simulink model "generic_20231123_1032"  (R2022b)
settings: Solver=ode45  StartTime=0.0  StopTime=50  RelTol=1e-3  EnableMultiTasking=on
model workspace (MAT data in the model file):
  A = 1
  B = 1.19071237887
  kd = -9.99955278144
  ki = 0.00519416981022
  kp = 9.99999979837
undefined symbols (not defined in the file): brake_select, curvature, DiscIntNeverNeededParam, speed
libraries: CarMaker4SL x88, simulink x1, mpcadaslib x1
(part 1 of 4)
settings Model: Creator=fh  LastModifiedBy=Admin
settings SolverCC: AlgebraicLoopSolver=TrustRegion
settings DataIOCC: LimitDataPoints=on  SaveFormat=Array  SignalLoggingSaveFormat=ModelDataLogs  ReturnWorkspaceOutputs=off  SignalLoggingName=sigsOut
settings OptimizationCC: BooleanDataType=off  ExpressionDepthLimit=2147483647  InitFltsAndDblsToZero=on  LifeSpan=inf
settings DebuggingCC: SaveWithParameterizedLinksMsg=none  UnderspecifiedInitializationDetection=Classic  MergeDetectMultiDrivingBlocksExec=none  SignalResolutionControl=TryResolveAllWithWarning  MultiTaskDSMMsg=warning  MultiTaskCondExecSysMsg=none  FcnCallInpInsideContextMsg=warning  UnconnectedInputMsg=warning  UnconnectedOutputMsg=warning  UnconnectedLineMsg=warning  StateNameClashWarn=warning  SFUnexpectedBacktrackingDiag=warning  SFNoUnconditionalDefaultTransitionDiag=warning  SFMachineParentedDataDiag=warning  ArithmeticOperatorsInVariantConditions=warning
settings HardwareCC: ProdBitPerPointer=32  ProdBitPerSizeT=32  ProdBitPerPtrDiffT=32  ProdLargestAtomicFloat=None  ProdIntDivRoundTo=Undefined  ProdEndianess=Unspecified  ProdWordSize=32  ProdHWDeviceType=32-bit Generic  TargetUnknown=on
settings ModelReferenceCC: EnableRefExpFcnMdlSchedulingChecks=on  PropagateSignalLabelsOutOfModel=off
settings SFSimCC: SimUseLocalCustomCode=off  CustomCodeUndefinedFunction=UseInterfaceOnly
settings RTWCC: RTWUseLocalCustomCode=off
settings CodeAppCC: MaxIdLength=63  StateflowObjectComments=on
settings GRTTargetCC: TargetFcnLib=ansi_tfl_tmw.mat  TargetLangStandard=C89/C90 (ANSI)  CombineOutputUpdateFcns=off  GRTInterface=on
settings ConfigComp: CovMetricSettings=dw  CovSaveCumulativeToWorkspaceVar=on  CovSaveSingleToWorkspaceVar=on  CovExternalEMLEnable=off

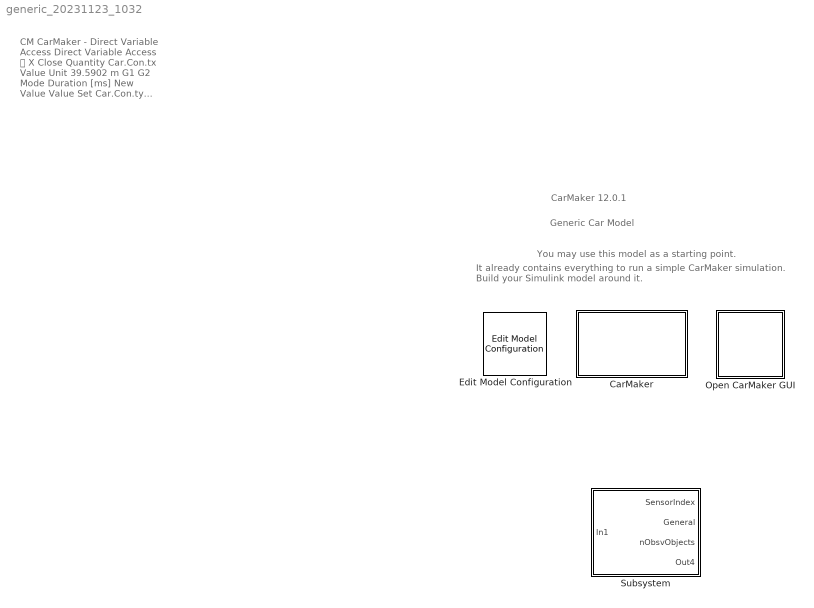
== system generic_20231123_1032 ==
  note: CM CarMaker - Direct Variable Access
      | Direct Variable Access
      | ப
      | X
      | Close
      | Quantity
      | Car.Con.tx
      | Value Unit 39.5902 m
      | G1 G2 Mode Duration [ms] New Value
      | Value
      | Set
      | Car.Con.ty
      | 503.638 m
      | Value
      | Set
      | Car.Con.tz
      | 12.6573 m
      | Value
      | Set
      | Car Road Path.DevAng
      | -0.0358446 rad
      | Value
      | Set
      | Car.Road.tx
      | 40.1728 m
      | Value
      | Set
      | Car Road.Path.DevDist
      | -0.152703 m
      | Ε
      | Value
      | Set
      | AccelCtrl.ACC.DesiredSpd
      | 31.2619 m/s
      | Value
      | Set
      | Sensor.Road.VehSensor_0.Path.tx
      | Sensor.Road.VehSensor_0.Path.ty
      | 0 m
      | Value
      | Set
      | 0 m
      | Value
      | Set
      | Sensor.Road.VehSensor_0.Path.tz
      | 0 m
      | Value
      | Set
      | Set Group 1
      | Set Group 2
      | Release all
  note: Generic Car Model
  note: You may use this model as a starting point.
  note: It already contains everything to run a simple CarMaker simulation.
      | Build your Simulink model around it.
  note: CarMaker 12.0.1
  CarMaker : Subsystem  TreatAsAtomicUnit=on
      mask Display: image(imread('CarMakerSys.png'));
  Edit Model Configuration : CarMaker4SL/Edit Model Configuration  SFunctionModules=''
  Open CarMaker GUI : Subsystem  LoadFcn=if ~length(which('cmself')), cmenv; end
      settings: OpenFcn=cmblockmagic('gui_fix_display'); CM_Simulink
      mask Display: image(imread('CarMakerGUI.png'));
  Subsystem : Subsystem

== system generic_20231123_1032/CarMaker ==
  CM_FIRST : Subsystem
  CM_LAST : Subsystem
  DrivMan : Subsystem
  Ground : Ground
  IPG Vehicle : Subsystem
  Terminator : Terminator
  VehicleControl : Subsystem
  wires:
  DrivMan/2(DrivMan.Out) -> VehicleControl/2(DrivMan.In)
  DrivMan/1(Sync_Out) -> VehicleControl/1(Sync_In)
  CM_FIRST/2(Env.Misc) -> DrivMan/2(Env.Misc)
  CM_FIRST/1(Sync_Out) -> DrivMan/1(Sync_In)
  CM_LAST/1(Sync_Out) -> Terminator/1
  Ground/1 -> CM_FIRST/1(Sync_In)
  IPG Vehicle/1(Sync_Out) -> CM_LAST/1(Sync_In)
  VehicleControl/1(Sync_Out) -> IPG Vehicle/1(Sync_In)
  VehicleControl/3(VhclCtrl.Steering) -> IPG Vehicle/3(VhclCtrl.Steering)
  VehicleControl/4(Vhcl.Wheel.In) -> IPG Vehicle/4(Vhcl.Wheel.In)
  VehicleControl/5(Vhcl.Misc) -> IPG Vehicle/5(Vhcl.Misc)
  VehicleControl/6(VhclCtrl.Brake) -> IPG Vehicle/6(VhclCtrl.Brake)
  VehicleControl/7(VhclCtrl.PT) -> IPG Vehicle/7(VhclCtrl.PT)
  VehicleControl/2(Vhcl.Model.Source) -> IPG Vehicle/2(Vhcl.Model.Source)

== system generic_20231123_1032/Open CarMaker GUI ==
  S-Function : S-Function  FunctionName=cm_gui  SFunctionDeploymentMode=off  EnableBusSupport=off

== system generic_20231123_1032/Subsystem ==
  In1 : Inport
  ADASRP Receive : CarMaker4SL/ADASRP Receive  Commented=on  xstime=Continuous
      settings: SourceProductName=CarMaker4SL
  Bus Selector : BusSelector  Commented=on  OutputSignals=ObjID,Type,DrvOn,LengthRear,LengthFront,Width,tPathOff,InDrvDir,nObjF,nObjR
  Bus Selector1 : BusSelector  Commented=on  OutputSignals=DistToLeftBorder,DistToRightBorder
  Constant : Constant  Commented=on  Value=0
  Constant1 : Constant  Commented=on  Value=0
  Object Sensor : CarMaker4SL/Sensors/Object Sensor  Commented=on  xname=0  xstime=Inherited
      settings: SourceProductName=CarMaker4SL
  Radar Sensor : CarMaker4SL/Sensors/Radar Sensor  Commented=on  xname=0  xstime=Continuous
      settings: SourceProductName=CarMaker4SL
  Scope : Scope  Commented=on  NumInputPorts=2
  Scope1 : Scope  Commented=on
  Scope2 : Scope  Commented=on  NumInputPorts=10
  SensorIndex : Outport
  General : Outport  Port=2
  nObsvObjects : Outport  Port=3
  Out4 : Outport  Port=4
  wires:
  Bus Selector/6 -> Scope2/6  "<Width>"
  Object Sensor/4 -> Scope1/1
  Bus Selector1/2 -> Scope/2  "<DistToRightBorder>"
  Radar Sensor/2 -> Bus Selector1/1
  Bus Selector/2 -> Scope2/2  "<Type>"
  Constant/1 -> Object Sensor/1
  Bus Selector/1 -> Scope2/1  "<ObjID>"
  Object Sensor/3 -> nObsvObjects/1
  Bus Selector/8 -> Scope2/8  "<InDrvDir>"
  Bus Selector/5 -> Scope2/5  "<LengthFront>"
  Constant1/1 -> Radar Sensor/1
  Bus Selector/10 -> Scope2/10  "<nObjR>"
  Bus Selector/9 -> Scope2/9  "<nObjF>"
  Bus Selector/4 -> Scope2/4  "<LengthRear>"
  Bus Selector1/1 -> Scope/1  "<DistToLeftBorder>"
  Bus Selector/7 -> Scope2/7  "<tPathOff>"
  Bus Selector/3 -> Scope2/3  "<DrvOn>"
  Object Sensor/2 -> General/1
  Object Sensor/1 -> SensorIndex/1
  In1/1 -> Bus Selector/1
  Radar Sensor/1 -> Out4/1

== system generic_20231123_1032/CarMaker/CM_FIRST ==
  Sync_In : Inport
  BusCreator1 : BusCreator  Inputs=8
  BusCreator2 : BusCreator  Inputs=6
  Demux1 : Demux  Outputs=14
      settings: DisplayOption=none
  Environment : S-Function  FunctionName=CM_Sfun  Parameters='Environment'  SFunctionDeploymentMode=off  EnableBusSupport=off
  IoIn : S-Function  FunctionName=CM_Sfun  Parameters='IoIn'  SFunctionDeploymentMode=off  EnableBusSupport=off
  Terminator : Terminator
  Sync_Out : Outport  VectorParamsAs1DForOutWhenUnconnected=off
  Env.Misc : Outport  Port=2  VectorParamsAs1DForOutWhenUnconnected=off
  wires:
  BusCreator2/1 -> Terminator/1  "IF Environment (in)"
  BusCreator1/1 -> Env.Misc/1
  Demux1/14 -> BusCreator2/6  "Env sRoad"
  Demux1/13 -> BusCreator2/5  "Env PoI_GCS Elev"
  Demux1/12 -> BusCreator2/4  "Env PoI_GCS Lat"
  Demux1/11 -> BusCreator2/3  "Env PoI_GCS Long"
  Demux1/10 -> BusCreator2/2  "Env Time"
  Demux1/9 -> BusCreator2/1  "Env yDay"
  Demux1/8 -> BusCreator1/8  "Env WindVel_tot z"
  Demux1/7 -> BusCreator1/7  "Env WindVel_tot y"
  Demux1/6 -> BusCreator1/6  "Env WindVel_tot x"
  Demux1/5 -> BusCreator1/5  "Env SolarRadiation"
  Demux1/4 -> BusCreator1/4  "Env AirHumidity"
  Demux1/3 -> BusCreator1/3  "Env AirPressure"
  Demux1/2 -> BusCreator1/2  "Env AirDensity"
  Demux1/1 -> BusCreator1/1  "Env Temperature"
  Environment/2 -> Demux1/1
  Environment/1 -> Sync_Out/1
  IoIn/1 -> Environment/1
  Sync_In/1 -> IoIn/1

== system generic_20231123_1032/CarMaker/CM_LAST ==
  Sync_In : Inport
  CM_User : S-Function  FunctionName=CM_Sfun  Parameters='CM_User'  SFunctionDeploymentMode=off  EnableBusSupport=off
  IoOut : S-Function  FunctionName=CM_Sfun  Parameters='IoOut'  SFunctionDeploymentMode=off  EnableBusSupport=off
  Sync_Out : Outport  VectorParamsAs1DForOutWhenUnconnected=off
  wires:
  IoOut/1 -> Sync_Out/1
  CM_User/1 -> IoOut/1
  Sync_In/1 -> CM_User/1

== system generic_20231123_1032/CarMaker/DrivMan ==
  note: There's rarely a reason to override DrivMan signals.
      | Use the VehicleControl interface for this purpose.
  Sync_In : Inport
  Env.Misc : Inport  Port=2
  BusCreator : BusCreator  Inputs=17
  Demux : Demux  Outputs=17
      settings: DisplayOption=none
  DrivMan : S-Function  FunctionName=CM_Sfun  Parameters='DrivMan'  SFunctionDeploymentMode=off  EnableBusSupport=off
  Sync_Out : Outport  VectorParamsAs1DForOutWhenUnconnected=off
  DrivMan.Out : Outport  Port=2  VectorParamsAs1DForOutWhenUnconnected=off
  wires:
  Demux/17 -> BusCreator/17  "DrivMan Steering Trq"
  Demux/16 -> BusCreator/16  "DrivMan Steering AngAcc"
  Demux/15 -> BusCreator/15  "DrivMan Steering AngVel"
  Demux/14 -> BusCreator/14  "DrivMan Steering Ang"
  Demux/12 -> BusCreator/12  "DrivMan Clutch"
  Demux/11 -> BusCreator/11  "DrivMan BrakePark"
  Demux/10 -> BusCreator/10  "DrivMan Brake"
  Demux/9 -> BusCreator/9  "DrivMan GearNo"
  Demux/8 -> BusCreator/8  "DrivMan SelectorCtrl"
  Demux/7 -> BusCreator/7  "DrivMan UserSignal4"
  Demux/6 -> BusCreator/6  "DrivMan UserSignal3"
  Demux/5 -> BusCreator/5  "DrivMan UserSignal2"
  Demux/4 -> BusCreator/4  "DrivMan UserSignal1"
  Demux/3 -> BusCreator/3  "DrivMan UserSignal0"
  Demux/2 -> BusCreator/2  "DrivMan Key"
  Demux/1 -> BusCreator/1  "DrivMan SST"
  Env.Misc/1 -> DrivMan/2
  Sync_In/1 -> DrivMan/1
  DrivMan/1 -> Sync_Out/1
  BusCreator/1 -> DrivMan.Out/1
  DrivMan/2 -> Demux/1
  Demux/13 -> BusCreator/13  "DrivMan Gas"

== system generic_20231123_1032/CarMaker/IPG Vehicle ==
  Sync_In : Inport
  Vhcl.Model.Source : Inport  Port=2
  VhclCtrl.Steering : Inport  Port=3
  Vhcl.Wheel.In : Inport  Port=4
  Vhcl.Misc : Inport  Port=5
  VhclCtrl.Brake : Inport  Port=6
  VhclCtrl.PT : Inport  Port=7
  Brake : Subsystem
  CarAndTrailer : Subsystem
  PowerTrain : Subsystem
  Stop Simulation : Stop
  VehicleSource_BuiltIn : simulink/Logic and Bit Operations/Compare To Constant  relop=~=  const=1  OutDataTypeStr=boolean  ZeroCross=off
  Sync_Out : Outport  VectorParamsAs1DForOutWhenUnconnected=off
  wires:
  VhclCtrl.PT/1 -> PowerTrain/3(VhclCtrl.PT)
  Brake/1(Sync_Out) -> PowerTrain/1(Sync_In)
  CarAndTrailer/1(Sync_Out) -> Brake/1(Sync_In)
  CarAndTrailer/2(Brake.IF.In) -> Brake/2(Brake.IF.In)
  VhclCtrl.Brake/1 -> Brake/3(VhclCtrl.Brake)
  PowerTrain/1(Sync_Out) -> Sync_Out/1
  Vhcl.Misc/1 -> CarAndTrailer/4(Vhcl.Misc)
  Vhcl.Wheel.In/1 -> CarAndTrailer/3(Vhcl.Wheel.In)
  VhclCtrl.Steering/1 -> CarAndTrailer/2(VhclCtrl.Steering)
  Sync_In/1 -> CarAndTrailer/1(Sync_In)
  Vhcl.Model.Source/1 -> VehicleSource_BuiltIn/1
  VehicleSource_BuiltIn/1 -> Stop Simulation/1
  Brake/2(Vhcl.Wheel.PT) -> PowerTrain/2(Vhcl.Wheel.PT)

== system generic_20231123_1032/CarMaker/VehicleControl ==
  note: <Your model here>
  note: When implementing a vehicle control model,
      | be sure to add '-disablevehiclecontrol' to the command line arguments
      | in the CarMaker Model Configuration block.
      | Otherwise your model will possibly not see the original DrivMan signals
      | on its inputs, but those of a currently activated C-coded vehicle control model instead.
  Sync_In : Inport
  DrivMan.In : Inport  Port=2
  Bus Creator2 : BusCreator  Inputs=2
  CreateBus Vhcl.Misc : Subsystem
  CreateBus Vhcl.Wheel.In : Subsystem
  CreateBus VhclCtrl : Subsystem
  CreateBus VhclCtrl.PT : Subsystem
  CreateBus VhclCtrl.Steering : Subsystem
  Demux2 : Demux  Outputs=2
      settings: DisplayOption=none
  Estimate object diemnsions : Subsystem
  Object sensor : Subsystem
  Read CM Dict10 : CarMaker4SL/Read CM Dict  xname=Vhcl.v  xsync=off  xstime=Continuous
  Smoothing : Subsystem
  Stanley controller : Subsystem
  VehicleControl : S-Function  FunctionName=CM_Sfun  Parameters='VehicleControl'  SFunctionDeploymentMode=off  EnableBusSupport=off
  VehicleControlUpd : S-Function  FunctionName=CM_Sfun  Parameters='VehicleControlUpd'  SFunctionDeploymentMode=off  EnableBusSupport=off
  Sync_Out : Outport  VectorParamsAs1DForOutWhenUnconnected=off
  Vhcl.Model.Source : Outport  Port=2  VectorParamsAs1DForOutWhenUnconnected=off
  VhclCtrl.Steering : Outport  Port=3  VectorParamsAs1DForOutWhenUnconnected=off
  Vhcl.Wheel.In : Outport  Port=4  VectorParamsAs1DForOutWhenUnconnected=off
  Vhcl.Misc : Outport  Port=5  VectorParamsAs1DForOutWhenUnconnected=off
  VhclCtrl.Brake : Outport  Port=6  VectorParamsAs1DForOutWhenUnconnected=off
  VhclCtrl.PT : Outport  Port=7  VectorParamsAs1DForOutWhenUnconnected=off
  wires:
  CreateBus VhclCtrl/1(Out) -> VehicleControlUpd/2
  VehicleControl/2 -> CreateBus VhclCtrl/1(In)
  VehicleControlUpd/2 -> Vhcl.Model.Source/1
  VehicleControlUpd/4 -> CreateBus Vhcl.Wheel.In/1(In1)
  VehicleControlUpd/5 -> CreateBus Vhcl.Misc/1(In1)
  VehicleControlUpd/6 -> Demux2/1
  VehicleControlUpd/7 -> CreateBus VhclCtrl.PT/1(In1)
  VehicleControlUpd/3 -> CreateBus VhclCtrl.Steering/1(In1)
  CreateBus Vhcl.Misc/1(Out1) -> Vhcl.Misc/1
  CreateBus Vhcl.Wheel.In/1(Out1) -> Vhcl.Wheel.In/1
  DrivMan.In/1 -> VehicleControl/2
  VehicleControl/1 -> VehicleControlUpd/1
  Sync_In/1 -> VehicleControl/1
  CreateBus VhclCtrl.PT/1(Out1) -> VhclCtrl.PT/1
  Bus Creator2/1 -> VhclCtrl.Brake/1
  CreateBus VhclCtrl.Steering/1(Out1) -> VhclCtrl.Steering/1
  VehicleControlUpd/1 -> Sync_Out/1
  Read CM Dict10/1 -> Stanley controller/1(V)
  CreateBus VhclCtrl/2(Steering_angle) -> Stanley controller/2(Steering_angle)
  Stanley controller/1(steering) -> Smoothing/1(Signal_In)
  Demux2/1 -> Bus Creator2/1  "VhclCtrl Brake"
  Demux2/2 -> Bus Creator2/2  "VhclCtrl BrakePark"
  Stanley controller/2(steering1) -> ?
  Smoothing/1(Signal_Out) -> CreateBus VhclCtrl/2(string)

== system generic_20231123_1032/CarMaker/IPG Vehicle/Brake ==
  note: When replacing the entire braking system,
      | be sure to disable the IPG brake model by using the brake
      | model 'Model Manager off' in the vehicle GUI.
  note: <Your model here>
  Sync_In : Inport
  Brake.IF.In : Inport  Port=2
  VhclCtrl.Brake : Inport  Port=3
  Brake : S-Function  FunctionName=CM_Sfun  Parameters='Brake'  SFunctionDeploymentMode=off  EnableBusSupport=off
  BrakeUpd : S-Function  FunctionName=CM_Sfun  Parameters='BrakeUpd'  SFunctionDeploymentMode=off  EnableBusSupport=off
  BusCreator1 : BusCreator  Inputs=16
  CreateBus Vhcl.Wheel.PT : Subsystem
  Demux : Demux  Outputs=16
      settings: DisplayOption=none
  Sync_Out : Outport  VectorParamsAs1DForOutWhenUnconnected=off
  Vhcl.Wheel.PT : Outport  Port=2  VectorParamsAs1DForOutWhenUnconnected=off
  wires:
  Demux/16 -> BusCreator1/16  "Brake IF Trq_DriveSrc_trg d3"
  Demux/15 -> BusCreator1/15  "Brake IF Trq_DriveSrc_trg d2"
  Demux/14 -> BusCreator1/14  "Brake IF Trq_DriveSrc_trg d1"
  Demux/13 -> BusCreator1/13  "Brake IF Trq_DriveSrc_trg d0"
  Demux/12 -> BusCreator1/12  "Brake IF Trq_Reg_trg RR"
  Demux/11 -> BusCreator1/11  "Brake IF Trq_Reg_trg RL"
  Demux/10 -> BusCreator1/10  "Brake IF Trq_Reg_trg FR"
  Demux/9 -> BusCreator1/9  "Brake IF Trq_Reg_trg FL"
  Demux/8 -> BusCreator1/8  "Brake IF Trq_PB RR"
  Demux/7 -> BusCreator1/7  "Brake IF Trq_PB RL"
  Demux/6 -> BusCreator1/6  "Brake IF Trq_PB FR"
  Demux/5 -> BusCreator1/5  "Brake IF Trq_PB FL"
  Demux/4 -> BusCreator1/4  "Brake IF Trq_WB RR"
  Demux/3 -> BusCreator1/3  "Brake IF Trq_WB RL"
  Demux/2 -> BusCreator1/2  "Brake IF Trq_WB FR"
  Demux/1 -> BusCreator1/1  "Brake IF Trq_WB FL"
  Brake/2 -> Demux/1
  BusCreator1/1 -> BrakeUpd/2
  BrakeUpd/1 -> Sync_Out/1
  Brake/1 -> BrakeUpd/1  "Sync"
  Brake.IF.In/1 -> Brake/2
  VhclCtrl.Brake/1 -> Brake/3
  Sync_In/1 -> Brake/1
  BrakeUpd/2 -> CreateBus Vhcl.Wheel.PT/1(In)
  CreateBus Vhcl.Wheel.PT/1(Out) -> Vhcl.Wheel.PT/1

== system generic_20231123_1032/CarMaker/IPG Vehicle/CarAndTrailer ==
  Sync_In : Inport
  VhclCtrl.Steering : Inport  Port=2
  Vhcl.Wheel.In : Inport  Port=3
  Vhcl.Misc : Inport  Port=4
  CarAndTrailerUpd : Subsystem
  Forces : Subsystem
  Ground : Ground
  Kinematics : Subsystem
  Kinetics : Subsystem
  Steering : Subsystem
  Terminator : Terminator
  Terminator1 : Terminator
  Trailer : Subsystem
  Sync_Out : Outport  VectorParamsAs1DForOutWhenUnconnected=off
  Brake.IF.In : Outport  Port=2  VectorParamsAs1DForOutWhenUnconnected=off
  wires:
  Trailer/9(Car.Hitch.FrcTrq) -> CarAndTrailerUpd/9(Car.Hitch.FrcTrq)
  Trailer/8(Vhcl.Wheel.RR) -> CarAndTrailerUpd/8(Vhcl.Wheel.RR)
  Trailer/7(Vhcl.Wheel.RL) -> CarAndTrailerUpd/7(Vhcl.Wheel.RL)
  Trailer/6(Vhcl.Wheel.FR) -> CarAndTrailerUpd/6(Vhcl.Wheel.FR)
  Trailer/5(Vhcl.Wheel.FL) -> CarAndTrailerUpd/5(Vhcl.Wheel.FL)
  Trailer/4(Vhcl.PoI) -> CarAndTrailerUpd/4(Vhcl.PoI)
  Trailer/3(Vhcl.Motion) -> CarAndTrailerUpd/3(Vhcl.Motion)
  Trailer/2(Vhcl.Steering) -> CarAndTrailerUpd/2(Vhcl.Steering)
  Trailer/1(Sync_Out) -> CarAndTrailerUpd/1(Sync_In)
  CarAndTrailerUpd/2(Brake.IF.In) -> Brake.IF.In/1
  CarAndTrailerUpd/1(Sync_Out) -> Sync_Out/1
  Vhcl.Misc/1 -> Terminator1/1
  Vhcl.Wheel.In/1 -> Terminator/1
  Kinetics/6(WheelCarrier.Misc) -> Trailer/6(WheelCarrier.Misc)
  Kinetics/5(Car.Trq_T2W) -> Trailer/5(Car.Trq_T2W)
  Steering/2(Steer.IF) -> Kinematics/2(Steer.IF)
  Kinetics/4(Car.Fr1) -> Trailer/4(Car.Fr1)
  Kinetics/3(Car.Hitch) -> Trailer/3(Car.Hitch)
  Kinetics/2(Trailer.Load) -> Trailer/2(Trailer.Load)
  VhclCtrl.Steering/1 -> Steering/2(VhclCtrl.Steering)
  Sync_In/1 -> Steering/1(Sync_In)
  Steering/1(Sync_Out) -> Kinematics/1(Sync_In)
  Kinetics/1(Sync_Out) -> Trailer/1(Sync_In)
  Ground/1 -> CarAndTrailerUpd/10(Vhcl.Fr1A)
  Forces/11(FStabi_ext) -> Kinetics/11(FStabi_ext)
  Forces/10(FDamp_ext) -> Kinetics/10(FDamp_ext)
  Forces/9(FSpring_ext) -> Kinetics/9(FSpring_ext)
  Forces/8(TireRR_Out) -> Kinetics/8(TireRR.Out)
  Forces/7(TireRL_Out) -> Kinetics/7(TireRL.Out)
  Forces/6(TireFR_Out) -> Kinetics/6(TireFR.Out)
  Forces/5(TireFL_Out) -> Kinetics/5(TireFL.Out)
  Forces/4(Car.Load) -> Kinetics/4(Car.Load)
  Forces/2(Car.Virtual) -> Kinetics/2(Car.Virtual)
  Kinematics/6(lSpring) -> Forces/6(lSpring)
  Kinematics/7(vDamp) -> Forces/7(vDamp)
  Forces/3(Car.Aero) -> Kinetics/3(Car.Aero)
  Forces/1(Sync_Out) -> Kinetics/1(Sync_In)
  Kinematics/5(TireRR_In) -> Forces/5(TireRR_In)
  Kinematics/4(TireRL_In) -> Forces/4(TireRL_In)
  Kinematics/3(TireFR_In) -> Forces/3(TireFR_In)
  Kinematics/2(TireFL_In) -> Forces/2(TireFL_In)
  Kinematics/1(Sync_Out) -> Forces/1(Sync_In)
  Kinematics/8(lStabi) -> Forces/8(lStabi)
  Forces/12(FBuf_ext) -> Kinetics/12(FBuf_ext)
  Kinematics/9(lBuf) -> Forces/9(lBuf)

== system generic_20231123_1032/CarMaker/IPG Vehicle/PowerTrain ==
  note: When replacing the entire powertrain,
      | be sure to disable the IPG powertrain model by using the powertrain
      | model 'Model Manager off' in the vehicle GUI.
  note: <Your model here>
  Sync_In : Inport
  Vhcl.Wheel.PT : Inport  Port=2
  VhclCtrl.PT : Inport  Port=3
  BusCreator1 : BusCreator  Inputs=42
  Demux1 : Demux  Outputs=42
      settings: DisplayOption=none
  PowerTrain : S-Function  FunctionName=CM_Sfun  Parameters='PowerTrain'  SFunctionDeploymentMode=off  EnableBusSupport=off
  PowerTrainUpd : S-Function  FunctionName=CM_Sfun  Parameters='PowerTrainUpd'  SFunctionDeploymentMode=off  EnableBusSupport=off
  Sync_Out : Outport  VectorParamsAs1DForOutWhenUnconnected=off
  wires:
  BusCreator1/1 -> PowerTrainUpd/2
  Demux1/42 -> BusCreator1/42  "PT IF WRR Trq_BrakeReg_max"
  Demux1/41 -> BusCreator1/41  "PT IF WRR Trq_BrakeReg"
  Demux1/40 -> BusCreator1/40  "PT IF WRR Trq_Supp2WC"
  Demux1/39 -> BusCreator1/39  "PT IF WRR Trq_Drive"
  Demux1/38 -> BusCreator1/38  "PT IF WRR Trq_B2W"
  Demux1/37 -> BusCreator1/37  "PT IF WRR rotv"
  Demux1/36 -> BusCreator1/36  "PT IF WRR rot"
  Demux1/35 -> BusCreator1/35  "PT IF WRL Trq_BrakeReg_max"
  Demux1/34 -> BusCreator1/34  "PT IF WRL Trq_BrakeReg"
  Demux1/33 -> BusCreator1/33  "PT IF WRL Trq_Supp2WC"
  Demux1/32 -> BusCreator1/32  "PT IF WRL Trq_Drive"
  Demux1/31 -> BusCreator1/31  "PT IF WRL Trq_B2W"
  Demux1/30 -> BusCreator1/30  "PT IF WRL rotv"
  Demux1/29 -> BusCreator1/29  "PT IF WRL rot"
  Demux1/28 -> BusCreator1/28  "PT IF WFR Trq_BrakeReg_max"
  Demux1/27 -> BusCreator1/27  "PT IF WFR Trq_BrakeReg"
  Demux1/26 -> BusCreator1/26  "PT IF WFR Trq_Supp2WC"
  Demux1/25 -> BusCreator1/25  "PT IF WFR Trq_Drive"
  Demux1/24 -> BusCreator1/24  "PT IF WFR Trq_B2W"
  Demux1/23 -> BusCreator1/23  "PT IF WFR rotv"
  Demux1/22 -> BusCreator1/22  "PT IF WFR rot"
  Demux1/21 -> BusCreator1/21  "PT IF WFL Trq_BrakeReg_max"
  Demux1/20 -> BusCreator1/20  "PT IF WFL Trq_BrakeReg"
  Demux1/19 -> BusCreator1/19  "PT IF WFL Trq_Supp2WC"
  Demux1/18 -> BusCreator1/18  "PT IF WFL Trq_Drive"
  Demux1/17 -> BusCreator1/17  "PT IF WFL Trq_B2W"
  Demux1/16 -> BusCreator1/16  "PT IF WFL rotv"
  Demux1/15 -> BusCreator1/15  "PT IF WFL rot"
  Demux1/14 -> BusCreator1/14  "PT IF DL_iDiff_mean"
  Demux1/13 -> BusCreator1/13  "PT IF Trq_Supp2BdyEng y"
  Demux1/12 -> BusCreator1/12  "PT IF Trq_Supp2BdyEng x"
  Demux1/11 -> BusCreator1/11  "PT IF Trq_Supp2Bdy1B z"
  Demux1/10 -> BusCreator1/10  "PT IF Trq_Supp2Bdy1B y"
  Demux1/9 -> BusCreator1/9  "PT IF Trq_Supp2Bdy1B x"
  Demux1/8 -> BusCreator1/8  "PT IF Trq_Supp2Bdy1 z"
  Demux1/7 -> BusCreator1/7  "PT IF Trq_Supp2Bdy1 y"
  Demux1/6 -> BusCreator1/6  "PT IF Trq_Supp2Bdy1 x"
  Demux1/5 -> BusCreator1/5  "PT IF Engine_rotv"
  Demux1/4 -> BusCreator1/4  "PT IF GearNo"
  Demux1/3 -> BusCreator1/3  "PT IF OperationError"
  Demux1/2 -> BusCreator1/2  "PT IF OperationState"
  Demux1/1 -> BusCreator1/1  "PT IF Ignition"
  Sync_In/1 -> PowerTrain/1
  PowerTrain/2 -> Demux1/1
  PowerTrainUpd/1 -> Sync_Out/1
  PowerTrain/1 -> PowerTrainUpd/1  "Sync"
  VhclCtrl.PT/1 -> PowerTrain/3
  Vhcl.Wheel.PT/1 -> PowerTrain/2

== system generic_20231123_1032/CarMaker/VehicleControl/CreateBus Vhcl.Misc ==
  In1 : Inport
  BusCreator : BusCreator  Inputs=11
  Demux : Demux  Outputs=11
      settings: DisplayOption=none
  Out1 : Outport  VectorParamsAs1DForOutWhenUnconnected=off
  wires:
  Demux/11 -> BusCreator/11  "Vhcl Wind_vel_0 z"
  Demux/10 -> BusCreator/10  "Vhcl Wind_vel_0 y"
  Demux/9 -> BusCreator/9  "Vhcl Wind_vel_0 x"
  Demux/8 -> BusCreator/8  "Vhcl Trq_DL2BdyEng y"
  Demux/7 -> BusCreator/7  "Vhcl Trq_DL2BdyEng x"
  Demux/6 -> BusCreator/6  "Vhcl Trq_DL2Bdy1B z"
  Demux/5 -> BusCreator/5  "Vhcl Trq_DL2Bdy1B y"
  Demux/4 -> BusCreator/4  "Vhcl Trq_DL2Bdy1B x"
  Demux/3 -> BusCreator/3  "Vhcl Trq_DL2Bdy1 z"
  Demux/2 -> BusCreator/2  "Vhcl Trq_DL2Bdy1 y"
  Demux/1 -> BusCreator/1  "Vhcl Trq_DL2Bdy1 x"
  In1/1 -> Demux/1
  BusCreator/1 -> Out1/1

== system generic_20231123_1032/CarMaker/VehicleControl/CreateBus Vhcl.Wheel.In ==
  In1 : Inport
  Bus Creator1 : BusCreator  Inputs=12
  Demux1 : Demux  Outputs=12
      settings: DisplayOption=none
  Display : Display
  Gain : Gain  Gain=0.309
  Out1 : Outport  VectorParamsAs1DForOutWhenUnconnected=off
  wires:
  Demux1/12 -> Bus Creator1/12  "Vhcl Wheel RR rotv"
  Demux1/11 -> Bus Creator1/11  "Vhcl Wheel RR Trq_DL2WC"
  Demux1/10 -> Bus Creator1/10  "Vhcl Wheel RR Trq_B2WC"
  Demux1/9 -> Bus Creator1/9  "Vhcl Wheel RL rotv"
  Demux1/8 -> Bus Creator1/8  "Vhcl Wheel RL Trq_DL2WC"
  Demux1/7 -> Bus Creator1/7  "Vhcl Wheel RL Trq_B2WC"
  Demux1/6 -> Bus Creator1/6  "Vhcl Wheel FR rotv"
  Demux1/5 -> Bus Creator1/5  "Vhcl Wheel FR Trq_DL2WC"
  Demux1/4 -> Bus Creator1/4  "Vhcl Wheel FR Trq_B2WC"
  Demux1/3 -> Bus Creator1/3  "Vhcl Wheel FL rotv"
  In1/1 -> Demux1/1
  Bus Creator1/1 -> Out1/1
  Demux1/2 -> Bus Creator1/2  "Vhcl Wheel FL Trq_DL2WC"
  Demux1/1 -> Bus Creator1/1  "Vhcl Wheel FL Trq_B2WC"
  Gain/1 -> Display/1

== system generic_20231123_1032/CarMaker/VehicleControl/CreateBus VhclCtrl ==
  In : Inport
  string : Inport  Port=2
  A*algoithm : Subsystem  Commented=on
  BusCreator : BusCreator  Inputs=29
  Demux : Demux  Outputs=29
      settings: DisplayOption=none
  Derivative : Derivative  Commented=on
  MATLAB Function : MATLAB Function  Commented=on  TreatAsAtomicUnit=on
  MATLAB Function1 : MATLAB Function  Commented=on  TreatAsAtomicUnit=on
  Read CM Dict2 : CarMaker4SL/Read CM Dict  Commented=on  xname=Car.YawRate  xsync=off  xstime=Continuous
  Stanley_controller : Subsystem  Commented=on
  Subsystem : Subsystem  Commented=on
  Subsystem1 : Subsystem  Commented=on
  Subsystem2 : Subsystem  Commented=on
  Subsystem3 : Subsystem  Commented=on
  Subsystem4 : Subsystem  Commented=on
  path_planner_MATLAB : Subsystem  Commented=on
  Out : Outport  VectorParamsAs1DForOutWhenUnconnected=off
  Steering_angle : Outport  Port=2  VectorParamsAs1DForOutWhenUnconnected=off
  wires:
  Demux/2 -> BusCreator/2  "VhclCtrl Key"
  Demux/11 -> BusCreator/11  "VhclCtrl BrakePark"
  Read CM Dict2/1 -> Derivative/1
  Demux/7 -> BusCreator/7  "VhclCtrl UserSignal4"
  Subsystem1/1(<ty>) -> Subsystem3/2(y2)
  Subsystem1/2(<tx>) -> Subsystem3/3(x2)
  Demux/5 -> BusCreator/5  "VhclCtrl UserSignal2"
  MATLAB Function/1(path_out) -> Stanley_controller/1(Path Out)
  Demux/9 -> BusCreator/9  "VhclCtrl SelectorCtrl"
  Derivative/1 -> Stanley_controller/2(Yaw_re)
  In/1 -> Demux/1
  Subsystem4/1(y_added) -> Subsystem2/1(In1)
  Demux/1 -> BusCreator/1  "VhclCtrl SST"
  Demux/3 -> BusCreator/3  "VhclCtrl UserSignal0"
  Demux/16 -> BusCreator/16  "VhclCtrl Steering AngAcc"
  Demux/4 -> BusCreator/4  "VhclCtrl UserSignal1"
  Demux/6 -> BusCreator/6  "VhclCtrl UserSignal3"
  Demux/8 -> BusCreator/8  "VhclCtrl GearNo"
  Demux/12 -> BusCreator/12  "VhclCtrl Clutch"
  Demux/15 -> BusCreator/15  "VhclCtrl Steering AngVel"
  Demux/17 -> BusCreator/17  "VhclCtrl Steering Trq"
  Demux/18 -> BusCreator/18  "VhclCtrl Lights LowBeam"
  Demux/19 -> BusCreator/19  "VhclCtrl Lights HighBeam"
  Demux/20 -> BusCreator/20  "VhclCtrl Lights Daytime"
  Demux/21 -> BusCreator/21  "VhclCtrl Lights ParkL"
  Demux/22 -> BusCreator/22  "VhclCtrl Lights ParkR"
  Demux/23 -> BusCreator/23  "VhclCtrl Lights IndL"
  Demux/24 -> BusCreator/24  "VhclCtrl Lights IndR"
  Demux/25 -> BusCreator/25  "VhclCtrl Lights FogFrontL"
  Demux/26 -> BusCreator/26  "VhclCtrl Lights FogFrontR"
  Demux/27 -> BusCreator/27  "VhclCtrl Lights FogRear"
  Demux/28 -> BusCreator/28  "VhclCtrl Lights Brake"
  Demux/29 -> BusCreator/29  "VhclCtrl Lights Reverse"
  BusCreator/1 -> Out/1
  Demux/13 -> BusCreator/13  "VhclCtrl Gas"
  Demux/14 -> BusCreator/14  "VhclCtrl Steering Ang"
  Subsystem/1(Out1) -> ?
  Subsystem/2(Out2) -> ?
  Subsystem/3(Out3) -> ?
  Demux/10 -> BusCreator/10  "VhclCtrl Brake"

== system generic_20231123_1032/CarMaker/VehicleControl/CreateBus VhclCtrl.PT ==
  In1 : Inport
  BusCreator1 : BusCreator  Inputs=12
  Demux1 : Demux  Outputs=12
      settings: DisplayOption=none
  Out1 : Outport  VectorParamsAs1DForOutWhenUnconnected=off
  wires:
  Demux1/12 -> BusCreator1/12  "VhclCtrl Brake"
  Demux1/11 -> BusCreator1/11  "VhclCtrl Gas"
  Demux1/10 -> BusCreator1/10  "VhclCtrl Clutch"
  Demux1/9 -> BusCreator1/9  "VhclCtrl SelectorCtrl"
  Demux1/8 -> BusCreator1/8  "VhclCtrl GearNo"
  Demux1/7 -> BusCreator1/7  "VhclCtrl UserSignal4"
  Demux1/6 -> BusCreator1/6  "VhclCtrl UserSignal3"
  Demux1/5 -> BusCreator1/5  "VhclCtrl UserSignal2"
  Demux1/4 -> BusCreator1/4  "VhclCtrl UserSignal1"
  Demux1/3 -> BusCreator1/3  "VhclCtrl UserSignal0"
  Demux1/2 -> BusCreator1/2  "VhclCtrl Key"
  Demux1/1 -> BusCreator1/1  "VhclCtrl SST"
  In1/1 -> Demux1/1
  BusCreator1/1 -> Out1/1

== system generic_20231123_1032/CarMaker/VehicleControl/CreateBus VhclCtrl.Steering ==
  note: Sensor.Object.RadarL.DrvLaneCurv
      | Sensor.Object.RadarL.relvTgt.dtct
      | Sensor.Object.RadarL.relvTgt.NearPnt.alpha
      | Sensor.Object.RadarL.relvTgt.NearPnt.ds.x
      | Sensor.Object.RadarL.relvTgt.NearPnt.ds.y
      | Sensor.Object.RadarL.relvTgt.NearPnt.ds.z
      | Sensor.Object.RadarL.relvTgt.NearPnt.ds_p
      | Sensor.Object.RadarL.relvTgt.NearPnt.dv.x
      | Sensor.Object.RadarL.relvTgt.NearPnt.dv.y
      | Sensor.Object.RadarL.relvTgt.RefPnt.ds.x
      | Sensor.Object.RadarL.relvTgt.RefPnt.ds.y
      | Sensor.Object.RadarL.relvTgt.RefPnt.dv.x
      | Sensor.Object.RadarL.relvTgt.RefPnt.r_zyx.x
      | Sensor.Object.RadarL.relvTgt.RefPnt.r_zyx.y
      | Sensor.Object.RadarL.relvTgt.RefPnt.dv_p
  In1 : Inport
  Bus Creator : BusCreator  Inputs=5
  Demux : Demux  Outputs=5
      settings: DisplayOption=none
  Display : Display  Commented=on
  MATLAB Function1 : MATLAB Function  Commented=on  TreatAsAtomicUnit=on
  MATLAB Function2 : MATLAB Function  Commented=on  TreatAsAtomicUnit=on
  Read CM Dict : CarMaker4SL/Read CM Dict  Commented=on  xname=Car.Road.Path.DevDist  xsync=off  xstime=Continuous
  Read CM Dict10 : CarMaker4SL/Read CM Dict  Commented=on  xname=Car.Con.tx  xsync=off  xstime=Continuous
  Read CM Dict11 : CarMaker4SL/Read CM Dict  Commented=on  xname=Car.Con.ty  xsync=off  xstime=Continuous
  Read CM Dict2 : CarMaker4SL/Read CM Dict  Commented=on  xname=Sensor.Object.RadarL.relvTgt.NearPnt.ds.x  xsync=off  xstime=Continuous
  Read CM Dict3 : CarMaker4SL/Read CM Dict  Commented=on  xname=Sensor.Object.RadarL.relvTgt.NearPnt.ds.y  xsync=off  xstime=Continuous
  Read CM Dict4 : CarMaker4SL/Read CM Dict  Commented=on  xname=Sensor.Object.RadarL.relvTgt.NearPnt.ds_p  xsync=off  xstime=Continuous
  Read CM Dict5 : CarMaker4SL/Read CM Dict  Commented=on  xname=Sensor.Object.RadarL.relvTgt.NearPnt.dv.x  xsync=off  xstime=Continuous
  Read CM Dict6 : CarMaker4SL/Read CM Dict  Commented=on  xname=Sensor.Object.RadarL.relvTgt.RefPnt.r_zyx.x  xsync=off  xstime=Continuous
  Read CM Dict7 : CarMaker4SL/Read CM Dict  Commented=on  xname=Sensor.Object.RadarL.relvTgt.RefPnt.r_zyx.y  xsync=off  xstime=Continuous
  Read CM Dict8 : CarMaker4SL/Read CM Dict  Commented=on  xname=Sensor.Object.RadarL.relvTgt.RefPnt.dv_p  xsync=off  xstime=Continuous
  Read CM Dict9 : CarMaker4SL/Read CM Dict  Commented=on  xname=Sensor.Camera.VehSensor_3.Obj.0.Type  xsync=off  xstime=Continuous
  Scope : Scope  NumInputPorts=3
  Scope1 : Scope  Commented=on  NumInputPorts=7
  Out1 : Outport  VectorParamsAs1DForOutWhenUnconnected=off
  wires:
  Bus Creator/1 -> Out1/1
  Demux/5 -> Bus Creator/5  "VhclCtrl Steering SteerByTrq"
  Demux/3 -> Bus Creator/3  "VhclCtrl Steering AngAcc"
  Demux/2 -> Bus Creator/2  "VhclCtrl Steering AngVel"
  Demux/4 -> Bus Creator/4  "VhclCtrl Steering Trq"
  Read CM Dict/1 -> MATLAB Function1/1(dev_dest)
  In1/1 -> Demux/1
  Read CM Dict2/1 -> Scope1/2
  Read CM Dict3/1 -> MATLAB Function2/4(trgt_y), MATLAB Function1/3(Y_dev), Scope1/1
  Read CM Dict4/1 -> MATLAB Function2/3(trgt_x), MATLAB Function1/2(y_car), Scope1/3
  Read CM Dict5/1 -> Scope1/4
  Read CM Dict6/1 -> Scope1/5
  Read CM Dict7/1 -> Scope1/6
  Read CM Dict8/1 -> Scope1/7  "Sensor.Object.RadarL.relvTgt.RefPnt.dv_p"
  Read CM Dict9/1 -> ?
  Read CM Dict11/1 -> MATLAB Function2/2(y_car)
  Read CM Dict10/1 -> MATLAB Function2/1(x_car)
  MATLAB Function2/1(nw_pth_gtd) -> Display/1
  Demux/1 -> Bus Creator/1  "VhclCtrl Steering Ang"

== system generic_20231123_1032/CarMaker/VehicleControl/Estimate object diemnsions ==
  note: % Example usage
      | range = 30;  % Replace with the actual range from your sensor
      | azimuth = deg2rad(10);  % Replace with the actual azimuth from your sensor
      | elevation = deg2rad(5);  % Replace with the actual elevation from your sensor
      | sensorFOV = [16, 8];  % Replace with the actual field of view of your sensor
      |
      | [estimatedWidth, estimatedHeight] = estimateObjectDimensions(range, azimuth, elevation, sensorFOV);
      |
      | disp(['Estimated Width: ', num2str(estimatedWidth), ' meters']);
      | disp(['Estimated Height: ', num2str(estimatedHeight), ' meters']);
  range : Inport
  azimuth : Inport  Port=2
  elevation : Inport  Port=3
  sensorFOV : Inport  Port=4
  sensorHeight : Inport  Port=5
  Constant1 : Constant  Commented=on  Value=16
  Constant2 : Constant  Commented=on  Value=8
  Constant4 : Constant  Commented=on  Value=0.309
  MATLAB Function : MATLAB Function  Commented=on  TreatAsAtomicUnit=on
  Mux : Mux  Commented=on  Inputs=2
  Read CM Dict2 : CarMaker4SL/Read CM Dict  Commented=on  xname=Sensor.Object.RadarL.relvTgt.RefPnt.r_zyx.y  xsync=off  xstime=Continuous
  Read CM Dict3 : CarMaker4SL/Read CM Dict  Commented=on  xname=Sensor.Object.RadarL.relvTgt.RefPnt.r_zyx.x  xsync=off  xstime=Continuous
  Read CM Dict4 : CarMaker4SL/Read CM Dict  Commented=on  xname=Sensor.Object.RadarL.Obj.T00.RefPnt.ds_p  xsync=off  xstime=Continuous
  Read CM Dict5 : CarMaker4SL/Read CM Dict  Commented=on  xname=Sensor.Object.RadarL.Obj.T00.RefPnt.ds.y  xsync=off  xstime=Continuous
  Read CM Dict6 : CarMaker4SL/Read CM Dict  Commented=on  xname=Sensor.Object.RadarL.Obj.T00.RefPnt.ds.x  xsync=off  xstime=Continuous
  Reshape : Reshape  Commented=on  OutputDimensionality=Customize  OutputDimensions=[1,2]
  Scope2 : Scope  Commented=on  NumInputPorts=3
  estimatedWidth : Outport
  estimatedHeight : Outport  Port=2
  Out3 : Outport  Port=3
  wires:
  sensorFOV/1 -> MATLAB Function/4(sensorFOV)
  Mux/1 -> Reshape/1
  MATLAB Function/1(estimatedWidth) -> estimatedWidth/1
  Constant1/1 -> Mux/1
  Read CM Dict6/1 -> Scope2/3
  MATLAB Function/2(estimatedHeight) -> estimatedHeight/1
  Constant2/1 -> Mux/2
  elevation/1 -> MATLAB Function/3(elevation)
  Read CM Dict5/1 -> Scope2/2
  Read CM Dict4/1 -> Scope2/1
  range/1 -> MATLAB Function/1(range)
  azimuth/1 -> MATLAB Function/2(azimuth)
  Reshape/1 -> Out3/1
  sensorHeight/1 -> MATLAB Function/5(sensorHeight)

== system generic_20231123_1032/CarMaker/VehicleControl/Object sensor ==
  Constant : Constant  Value=0
  Object Sensor : CarMaker4SL/Sensors/Object Sensor  Commented=on  xname=0  xstime=Continuous
      settings: SourceProductName=CarMaker4SL
  Read CM Dict : CarMaker4SL/Read CM Dict  Commented=on  xname=Sensor.Object.RadarL.relvTgt.NearPnt.ds.x  xsync=off  xstime=Continuous
  Read CM Dict1 : CarMaker4SL/Read CM Dict  Commented=on  xname=Sensor.Object.RadarL.relvTgt.NearPnt.ds.y  xsync=off  xstime=Continuous
  Scope1 : Scope  Commented=on  NumInputPorts=2
  SensorIndex : Outport
  General : Outport  Port=2
  nObsvObjects : Outport  Port=3
  Target : Outport  Port=4
  wires:
  Object Sensor/2 -> General/1
  Constant/1 -> Object Sensor/1
  Read CM Dict/1 -> Scope1/1
  Read CM Dict1/1 -> Scope1/2
  Object Sensor/4 -> Target/1
  Object Sensor/1 -> SensorIndex/1
  Object Sensor/3 -> nObsvObjects/1

== system generic_20231123_1032/CarMaker/VehicleControl/Smoothing ==
  Signal_In : Inport
  Add : Sum  Inputs=++++
  Delay : Delay  InitialCondition=0.1
  Delay1 : Delay  DelayLength=4  InitialCondition=0.1
  Delay2 : Delay  DelayLength=5  InitialCondition=0.1
  Gain : Gain  Gain=0.35
  Gain1 : Gain  Gain=0.25
  Gain2 : Gain  Gain=0.25
  Gain3 : Gain  Gain=0.15
  Signal_Out : Outport  VectorParamsAs1DForOutWhenUnconnected=off
  wires:
  Gain1/1 -> Add/2
  Signal_In/1 -> Gain/1
  Delay/1 -> Gain1/1
  Gain/1 -> Add/1
  Delay1/1 -> Gain2/1
  Add/1 -> Delay2/1, Delay1/1, Delay/1, Signal_Out/1
  Gain2/1 -> Add/3
  Delay2/1 -> Gain3/1
  Gain3/1 -> Add/4

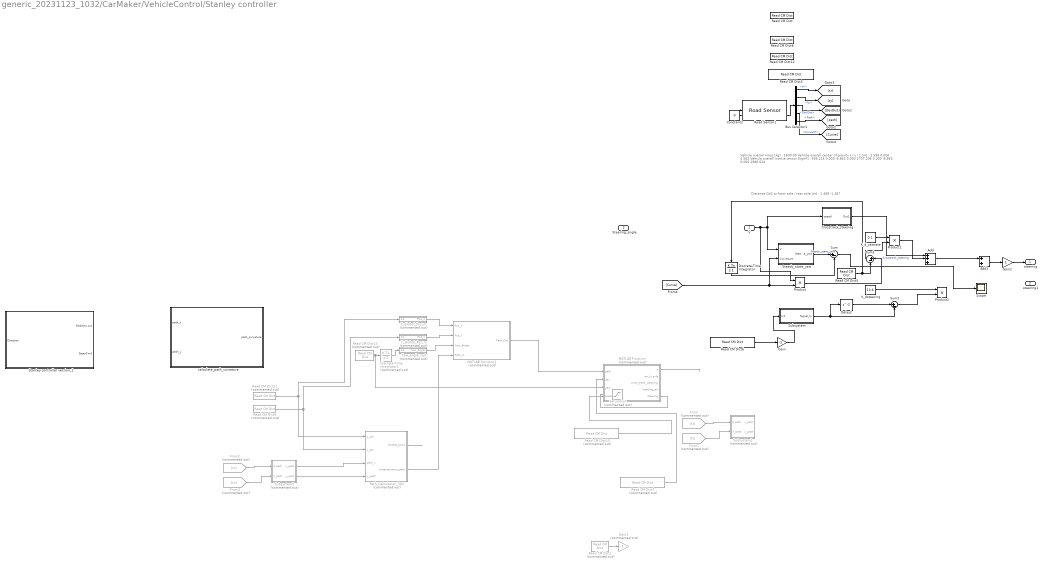
== system generic_20231123_1032/CarMaker/VehicleControl/Stanley controller ==
  note: Vehicle overall mass [kg] 	: 	1600.00
      |
      |  Vehicle overall center of gravity x / y / z [m] 	: 	2.596	0.000	0.562
      |
      |  Vehicle overall inertia tensor [kgm²] 	: 	696.215	0.000	-8.863
      |  	 									0.000	2707.206	0.000
      |  	 									-8.863	0.000	2986.624
  note: Distance CoG to front axle / rear axle [m] : 1.488 -1.487
  V : Inport
  Steering_angle : Inport  Port=2
  Add : Sum  Inputs=+++
  Add1 : Sum
  Bus Selector1 : BusSelector  OutputSignals=Path.tx,Path.ty,Path.DevDist,Path.CurveXY,Path
  Constant2 : Constant  Value=0
  Crosstrack_steering : Subsystem
  Delay2 : Delay
  Discrete-Time Integrator : DiscreteIntegrator  SampleTime=-1  ICPrevOutput=DiscIntNeverNeededParam  ICPrevScaledInput=DiscIntNeverNeededParam
  Discrete-Time Integrator1 : DiscreteIntegrator  Commented=on  SampleTime=-1  ICPrevOutput=DiscIntNeverNeededParam  ICPrevScaledInput=DiscIntNeverNeededParam
  From : From  Commented=on  GotoTag=tx
  From1 : From  Commented=on  GotoTag=ty
  From2 : From  Commented=on  GotoTag=tx
  From3 : From  Commented=on  GotoTag=ty
  Gain : Gain  Gain=-1
  Gain1 : Gain
  Gain3 : Gain  Commented=on  Gain=-1
  K_d_yawrate : Constant  Value=0.1
  K_dsteering : Constant  Value=13.6
  MATLAB Function : MATLAB Function  Commented=on  TreatAsAtomicUnit=on
  MATLAB Function1 : MATLAB Function  Commented=on  TreatAsAtomicUnit=on
  Path_Calculation_V02 : MATLAB Function  Commented=on  TreatAsAtomicUnit=on
  Product : Product
  Product1 : Product
  Product2 : Product
  Read CM Dict : CarMaker4SL/Read CM Dict  xname=Car.Road.Path.DevDist  xsync=off  xstime=Continuous
  Read CM Dict1 : CarMaker4SL/Read CM Dict  Commented=on  xname=Car.Yaw  xsync=off  xstime=Continuous
  Read CM Dict10 : CarMaker4SL/Read CM Dict  Commented=on  xname=Vhcl.v  xsync=off  xstime=Continuous
  Read CM Dict11 : CarMaker4SL/Read CM Dict  Commented=on  xname=Car.Gen.tx  xsync=off  xstime=Continuous
  Read CM Dict12 : CarMaker4SL/Read CM Dict  xname=Car.Gen.ty  xsync=off  xstime=Continuous
  Read CM Dict13 : CarMaker4SL/Read CM Dict  Commented=on  xname=Car.YawRate  xsync=off  xstime=Continuous
  Read CM Dict3 : CarMaker4SL/Read CM Dict  xname=Vhcl.Yaw  xsync=off  xstime=Continuous
  Read CM Dict5 : CarMaker4SL/Read CM Dict  xname=Car.YawRate  xsync=off  xstime=Continuous
  Read CM Dict6 : CarMaker4SL/Read CM Dict  xname=Car.Road.Path.DevDist  xsync=off  xstime=Continuous
  Read CM Dict7 : CarMaker4SL/Read CM Dict  Commented=on  xname=Car.Road.Path.DevDist  xsync=off  xstime=Continuous
  Read CM Dict8 : CarMaker4SL/Read CM Dict  xname=Car.Gen.tx  xsync=off  xstime=Continuous
  Read CM Dict9 : CarMaker4SL/Read CM Dict  Commented=on  xname=Car.Gen.ty  xsync=off  xstime=Continuous
  Road Sensor1 : CarMaker4SL/Sensors/Road Sensor  xname=0  xstime=Continuous
      settings: SourceProductName=CarMaker4SL
  Saturation : Saturate  Commented=on  UpperLimit=1.6  LowerLimit=-1.6
  Scope : Scope
  Stanley controller version_1 : Subsystem  Variant=on  VariantControlMode=label  VariantControl=Choice  LabelModeActiveChoice=Choice
  Steady_state_yaw : Subsystem
  Subsystem : Subsystem
  Subsystem1 : Subsystem  Commented=on
  Subsystem3 : Subsystem  Commented=on
  Sum : Sum  Inputs=|+-
  Sum1 : Sum  Inputs=|+-
  Sum2 : Sum  Inputs=|+-
  X_Global_Pos_m : Subsystem  Commented=on
  Y_Global_Pos_m : Subsystem  Commented=on
  Yaw_angle_rad : Subsystem  Commented=on
  calculate_path_curvature : MATLAB Function  TreatAsAtomicUnit=on
  steering : Outport
  steering1 : Outport  Port=2
  wires:
  Constant2/1 -> Road Sensor1/1
  Road Sensor1/2 -> Bus Selector1/1
  Bus Selector1/2 -> [ty]  "<ty>"
  Bus Selector1/3 -> [DevDist]  "<DevDist>"
  Bus Selector1/5 -> [path]  "<Path>"
  Bus Selector1/1 -> [tx]  "<tx>"
  Bus Selector1/4 -> [Curve]  "<CurveXY>"
  V/1 -> Product/1, Crosstrack_steering/1(speed), Steady_state_yaw/1(V)
  Steady_state_yaw/1(Steady_state_yaw) -> Sum/1  "Steady_state_yaw"
  [Curve] -> Steady_state_yaw/2(Curvature), Product/2
  Read CM Dict5/1 -> Discrete-Time Integrator/1, Sum1/2
  Product/1 -> Sum1/1
  Sum1/1 -> Product1/2
  K_d_yawrate/1 -> Product1/1
  Subsystem/1(Signal_In) -> Delay2/1, Sum2/2
  K_dsteering/1 -> Product2/1
  Discrete-Time Integrator/1 -> Sum/2
  Add1/1 -> Gain1/1
  Gain/1 -> Subsystem/1(In1)
  Read CM Dict6/1 -> Gain/1
  Add/1 -> Add1/1
  Product1/1 -> Add/2
  Crosstrack_steering/1(Out1) -> Add/1  "Crosstrack_steering"
  Sum/1 -> Scope/1
  Gain1/1 -> steering/1
  Delay2/1 -> Sum2/1
  Sum2/1 -> Product2/2
  From/1 -> Subsystem1/1(X-path)
  From1/1 -> Subsystem1/2(Y_path)
  Read CM Dict10/1 -> MATLAB Function/4(speed_act)
  MATLAB Function/5(steering) -> Saturation/1
  MATLAB Function/1(e) -> ?
  Read CM Dict11/1 -> X_Global_Pos_m/1(In1), Path_Calculation_V02/1(x_car)
  Read CM Dict9/1 -> Y_Global_Pos_m/1(In1), Path_Calculation_V02/2(y_car)
  Subsystem3/2(y_path) -> Path_Calculation_V02/4(y_path)
  From2/1 -> Subsystem3/1(X-path)
  Subsystem3/1(x_path) -> Path_Calculation_V02/3(path_x)
  From3/1 -> Subsystem3/2(Y_path)
  Path_Calculation_V02/1(closest_point) -> ?
  Read CM Dict1/1 -> Gain3/1
  Read CM Dict7/1 -> MATLAB Function/2(dev)
  Path_Calculation_V02/2(instantaneous_path) -> MATLAB Function1/4(Path_In)
  Read CM Dict13/1 -> MATLAB Function/3(yaw), Discrete-Time Integrator1/1
  Discrete-Time Integrator1/1 -> Yaw_angle_rad/1(In1)
  X_Global_Pos_m/1(Pos_X) -> MATLAB Function1/1(Pos_X)
  Y_Global_Pos_m/1(Pos_Y) -> MATLAB Function1/2(Pos_Y)
  Yaw_angle_rad/1(Yaw_Angle) -> MATLAB Function1/3(Yaw_Angle)
  MATLAB Function1/1(Path_Out) -> MATLAB Function/1(path)

== system generic_20231123_1032/CarMaker/IPG Vehicle/Brake/CreateBus Vhcl.Wheel.PT ==
  In : Inport
  BusCreator1 : BusCreator  Inputs=20
  Demux1 : Demux  Outputs=20
      settings: DisplayOption=none
  Out : Outport  VectorParamsAs1DForOutWhenUnconnected=off
  wires:
  Demux1/20 -> BusCreator1/20  "Vhcl Trq_DriveSrc_trg d3"
  Demux1/19 -> BusCreator1/19  "Vhcl Trq_DriveSrc_trg d2"
  Demux1/18 -> BusCreator1/18  "Vhcl Trq_DriveSrc_trg d1"
  Demux1/17 -> BusCreator1/17  "Vhcl Trq_DriveSrc_trg d0"
  Demux1/16 -> BusCreator1/16  "Vhcl Wheel RR WhlBearing"
  Demux1/15 -> BusCreator1/15  "Vhcl Wheel RR Trq_T2W"
  Demux1/14 -> BusCreator1/14  "Vhcl Wheel RR Trq_BrakeReg_trg"
  Demux1/13 -> BusCreator1/13  "Vhcl Wheel RR Trq_Brake"
  Demux1/12 -> BusCreator1/12  "Vhcl Wheel RL WhlBearing"
  Demux1/11 -> BusCreator1/11  "Vhcl Wheel RL Trq_T2W"
  Demux1/10 -> BusCreator1/10  "Vhcl Wheel RL Trq_BrakeReg_trg"
  Demux1/9 -> BusCreator1/9  "Vhcl Wheel RL Trq_Brake"
  Demux1/8 -> BusCreator1/8  "Vhcl Wheel FR WhlBearing"
  Demux1/7 -> BusCreator1/7  "Vhcl Wheel FR Trq_T2W"
  Demux1/6 -> BusCreator1/6  "Vhcl Wheel FR Trq_BrakeReg_trg"
  Demux1/5 -> BusCreator1/5  "Vhcl Wheel FR Trq_Brake"
  Demux1/4 -> BusCreator1/4  "Vhcl Wheel FL WhlBearing"
  Demux1/3 -> BusCreator1/3  "Vhcl Wheel FL Trq_T2W"
  Demux1/2 -> BusCreator1/2  "Vhcl Wheel FL Trq_BrakeReg_trg"
  Demux1/1 -> BusCreator1/1  "Vhcl Wheel FL Trq_Brake"
  BusCreator1/1 -> Out/1
  In/1 -> Demux1/1

== system generic_20231123_1032/CarMaker/IPG Vehicle/CarAndTrailer/CarAndTrailerUpd ==
  Sync_In : Inport
  Vhcl.Steering : Inport  Port=2
  Vhcl.Motion : Inport  Port=3
  Vhcl.PoI : Inport  Port=4
  Vhcl.Wheel.FL : Inport  Port=5
  Vhcl.Wheel.FR : Inport  Port=6
  Vhcl.Wheel.RL : Inport  Port=7
  Vhcl.Wheel.RR : Inport  Port=8
  Car.Hitch.FrcTrq : Inport  Port=9
  Vhcl.Fr1A : Inport  Port=10
  CarAndTrailerUpd : S-Function  FunctionName=CM_Sfun  Parameters='CarAndTrUpd'  SFunctionDeploymentMode=off  EnableBusSupport=off
  CreateBus Brake.IF.In : Subsystem
  Sync_Out : Outport  VectorParamsAs1DForOutWhenUnconnected=off
  Brake.IF.In : Outport  Port=2  VectorParamsAs1DForOutWhenUnconnected=off
  wires:
  Vhcl.Fr1A/1 -> CarAndTrailerUpd/10  "user vehicle only"
  Vhcl.Steering/1 -> CarAndTrailerUpd/2
  Vhcl.Motion/1 -> CarAndTrailerUpd/3
  Vhcl.PoI/1 -> CarAndTrailerUpd/4
  Vhcl.Wheel.FL/1 -> CarAndTrailerUpd/5
  Vhcl.Wheel.FR/1 -> CarAndTrailerUpd/6
  Car.Hitch.FrcTrq/1 -> CarAndTrailerUpd/9
  Vhcl.Wheel.RR/1 -> CarAndTrailerUpd/8
  Vhcl.Wheel.RL/1 -> CarAndTrailerUpd/7
  CarAndTrailerUpd/2 -> CreateBus Brake.IF.In/1(In)
  CreateBus Brake.IF.In/1(Out) -> Brake.IF.In/1
  CarAndTrailerUpd/1 -> Sync_Out/1
  Sync_In/1 -> CarAndTrailerUpd/1

== system generic_20231123_1032/CarMaker/IPG Vehicle/CarAndTrailer/Forces ==
  Sync_In : Inport
  TireFL_In : Inport  Port=2
  TireFR_In : Inport  Port=3
  TireRL_In : Inport  Port=4
  TireRR_In : Inport  Port=5
  lSpring : Inport  Port=6
  vDamp : Inport  Port=7
  lStabi : Inport  Port=8
  lBuf : Inport  Port=9
  External Suspension Forces : Subsystem
  Suspension Forces : Subsystem
  Tires : Subsystem
  Vehicle Forces : Subsystem
  Sync_Out : Outport  VectorParamsAs1DForOutWhenUnconnected=off
  Car.Virtual : Outport  Port=2  VectorParamsAs1DForOutWhenUnconnected=off
  Car.Aero : Outport  Port=3  VectorParamsAs1DForOutWhenUnconnected=off
  Car.Load : Outport  Port=4  VectorParamsAs1DForOutWhenUnconnected=off
  TireFL_Out : Outport  Port=5  VectorParamsAs1DForOutWhenUnconnected=off
  TireFR_Out : Outport  Port=6  VectorParamsAs1DForOutWhenUnconnected=off
  TireRL_Out : Outport  Port=7  VectorParamsAs1DForOutWhenUnconnected=off
  TireRR_Out : Outport  Port=8  VectorParamsAs1DForOutWhenUnconnected=off
  FSpring_ext : Outport  Port=9  VectorParamsAs1DForOutWhenUnconnected=off
  FDamp_ext : Outport  Port=10  VectorParamsAs1DForOutWhenUnconnected=off
  FStabi_ext : Outport  Port=11  VectorParamsAs1DForOutWhenUnconnected=off
  FBuf_ext : Outport  Port=12  VectorParamsAs1DForOutWhenUnconnected=off
  wires:
  lBuf/1 -> External Suspension Forces/5(lBuf), Suspension Forces/5(lBuf)
  lStabi/1 -> External Suspension Forces/4(lStabi), Suspension Forces/4(lStabi)
  vDamp/1 -> External Suspension Forces/3(vDamp), Suspension Forces/3(vDamp)
  Tires/4(TireRR_Out) -> TireRR_Out/1
  Tires/3(TireRL_Out) -> TireRL_Out/1
  Tires/2(TireFR_Out) -> TireFR_Out/1
  Tires/1(TireFL_Out) -> TireFL_Out/1
  TireRR_In/1 -> Tires/5(TireRR_In)
  TireRL_In/1 -> Tires/4(TireRL_In)
  TireFR_In/1 -> Tires/3(TireFR_In)
  TireFL_In/1 -> Tires/2(TireFL_In)
  External Suspension Forces/4(FBuf_ext) -> FBuf_ext/1
  Sync_In/1 -> External Suspension Forces/1(Sync_In), Tires/1(Sync_In), Vehicle Forces/1(Sync_In)
  Vehicle Forces/1(Sync_Out) -> Suspension Forces/1(Sync_In)
  Vehicle Forces/2(Car.Virtual) -> Car.Virtual/1
  Vehicle Forces/3(Car.Aero) -> Car.Aero/1
  Vehicle Forces/4(Car.Load) -> Car.Load/1
  lSpring/1 -> External Suspension Forces/2(lSpring), Suspension Forces/2(lSpring)
  External Suspension Forces/2(FDamp_ext) -> FDamp_ext/1
  External Suspension Forces/3(FStabi_ext) -> FStabi_ext/1
  External Suspension Forces/1(FSpring_ext) -> FSpring_ext/1
  Suspension Forces/1(Sync_Out) -> Sync_Out/1

== system generic_20231123_1032/CarMaker/IPG Vehicle/CarAndTrailer/Kinematics ==
  Sync_In : Inport
  Steer.IF : Inport  Port=2
  Kinematics : S-Function  FunctionName=CM_Sfun  Parameters='Kinematics'  SFunctionDeploymentMode=off  EnableBusSupport=off
  Sync_Out : Outport  VectorParamsAs1DForOutWhenUnconnected=off
  TireFL_In : Outport  Port=2  VectorParamsAs1DForOutWhenUnconnected=off
  TireFR_In : Outport  Port=3  VectorParamsAs1DForOutWhenUnconnected=off
  TireRL_In : Outport  Port=4  VectorParamsAs1DForOutWhenUnconnected=off
  TireRR_In : Outport  Port=5  VectorParamsAs1DForOutWhenUnconnected=off
  lSpring : Outport  Port=6  VectorParamsAs1DForOutWhenUnconnected=off
  vDamp : Outport  Port=7  VectorParamsAs1DForOutWhenUnconnected=off
  lStabi : Outport  Port=8  VectorParamsAs1DForOutWhenUnconnected=off
  lBuf : Outport  Port=9  VectorParamsAs1DForOutWhenUnconnected=off
  wires:
  Kinematics/9 -> lBuf/1
  Kinematics/8 -> lStabi/1
  Kinematics/2 -> TireFL_In/1
  Kinematics/3 -> TireFR_In/1
  Kinematics/4 -> TireRL_In/1
  Kinematics/5 -> TireRR_In/1
  Kinematics/6 -> lSpring/1
  Kinematics/7 -> vDamp/1
  Sync_In/1 -> Kinematics/1
  Kinematics/1 -> Sync_Out/1
  Steer.IF/1 -> Kinematics/2
